simulink library "helperVarsizeLib"  (R2022b)
settings: Solver=VariableStepAuto  StartTime=0.0  StopTime=10.0  RelTol=1e-3
settings Model: Creator=The MathWorks, Inc.  LastModifiedBy=The MathWorks, Inc.
settings SolverCC: AlgebraicLoopSolver=TrustRegion
settings DebuggingCC: UnconnectedInputMsg=warning  UnconnectedOutputMsg=warning  UnconnectedLineMsg=warning  SFMachineParentedDataDiag=warning  ArithmeticOperatorsInVariantConditions=warning
settings ModelReferenceCC: EnableRefExpFcnMdlSchedulingChecks=on
settings SFSimCC: CustomCodeUndefinedFunction=UseInterfaceOnly
settings RTWCC: DLArmComputeVersion=19.05

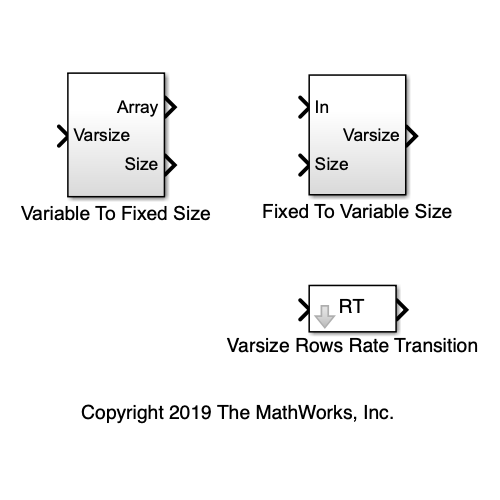
[thumbnail: Simulink's stored preview of the top-level diagram]
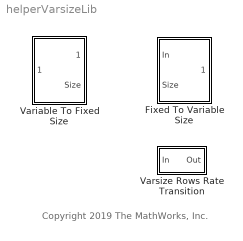
== system helperVarsizeLib ==
  note: Copyright 2019 The MathWorks, Inc.
  Fixed To Variable Size : Subsystem
  Variable To Fixed Size : Subsystem
  Varsize Rows Rate Transition : Subsystem  mask(Variable Size Rows Rate Transition){bufferInitialCondition=zeros(500,1)}
      mask prompts: bufferInitialCondition "Buffer initial condition"
      mask help: Helper block which enables rate transitions for arrays with variable sized rows. The maximium buffer size is the same as the buffer initial condition.
      mask Display: disp('RT')

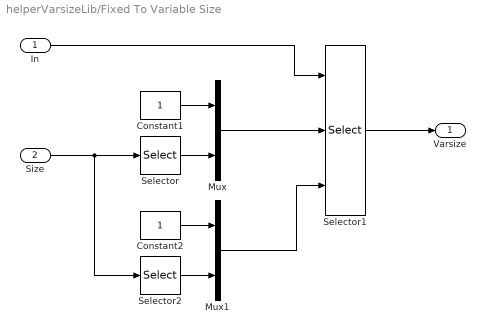
== system helperVarsizeLib/Fixed To Variable Size ==
  In : Inport
  Size : Inport  Port=2
  Constant1 : Constant  VectorParams1D=off
  Constant2 : Constant  VectorParams1D=off
  Mux : Mux  Inputs=2
  Mux1 : Mux  Inputs=2
  Selector : Selector  InputPortWidth=2  IndexOptions=Index vector (dialog)  Indices=1  OutputSizes=1
  Selector1 : Selector  NumberOfDimensions=2  InputPortWidth=3  IndexOptions=Starting and ending indices (port),Starting and ending indices (port)  Indices=[1 3],1  OutputSizes=1,1
  Selector2 : Selector  InputPortWidth=2  IndexOptions=Index vector (dialog)  Indices=2  OutputSizes=1
  Varsize : Outport  VectorParamsAs1DForOutWhenUnconnected=off
  wires:
  Constant2/1 -> Mux1/1
  Mux1/1 -> Selector1/3
  Selector2/1 -> Mux1/2
  Selector/1 -> Mux/2
  In/1 -> Selector1/1
  Selector1/1 -> Varsize/1
  Mux/1 -> Selector1/2
  Constant1/1 -> Mux/1
  Size/1 -> Selector/1, Selector2/1

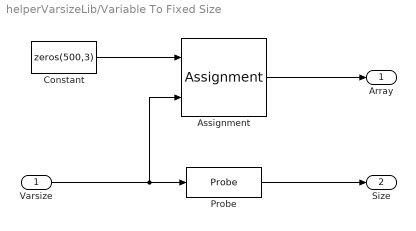
== system helperVarsizeLib/Variable To Fixed Size ==
  Varsize : Inport
  Assignment : Assignment  NumberOfDimensions=2  IndexMode=Zero-based  DiagnosticForDimensions=Warning  IndexOptions=Starting index (dialog),Starting index (dialog)  Indices=0,0  OutputSizes=1,1
  Constant : Constant  Value=zeros(500,3)  VectorParams1D=off
  Probe : Probe  ProbeWidth=off  ProbeSampleTime=off  ProbeComplexSignal=off  ProbeSignalDimensions=on
  Array : Outport  VectorParamsAs1DForOutWhenUnconnected=off
  Size : Outport  Port=2  VectorParamsAs1DForOutWhenUnconnected=off
  wires:
  Constant/1 -> Assignment/1
  Varsize/1 -> Probe/1, Assignment/2
  Assignment/1 -> Array/1
  Probe/1 -> Size/1

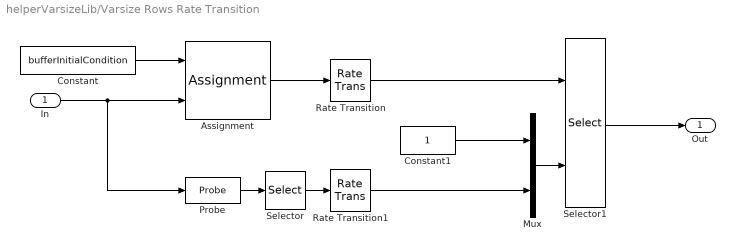
== system helperVarsizeLib/Varsize Rows Rate Transition ==
  In : Inport
  Assignment : Assignment  NumberOfDimensions=2  IndexMode=Zero-based  DiagnosticForDimensions=Warning  IndexOptions=Starting index (dialog),Starting index (dialog)  Indices=0,0  OutputSizes=1,1
  Constant : Constant  Value=bufferInitialCondition  VectorParams1D=off
  Constant1 : Constant  VectorParams1D=off
  Mux : Mux  Inputs=2
  Probe : Probe  ProbeWidth=off  ProbeSampleTime=off  ProbeComplexSignal=off  ProbeSignalDimensions=on
  Rate Transition : RateTransition  InitialCondition=bufferInitialCondition
  Rate Transition1 : RateTransition  InitialCondition=1
  Selector : Selector  InputPortWidth=2  IndexOptions=Index vector (dialog)  Indices=1  OutputSizes=1
  Selector1 : Selector  NumberOfDimensions=2  InputPortWidth=3  IndexOptions=Starting and ending indices (port),Select all  Indices=[1 3],1  OutputSizes=1,1
  Out : Outport  VectorParamsAs1DForOutWhenUnconnected=off
  wires:
  Selector/1 -> Rate Transition1/1
  In/1 -> Probe/1, Assignment/2
  Mux/1 -> Selector1/2
  Selector1/1 -> Out/1
  Assignment/1 -> Rate Transition/1
  Rate Transition/1 -> Selector1/1
  Constant1/1 -> Mux/1
  Constant/1 -> Assignment/1
  Probe/1 -> Selector/1
  Rate Transition1/1 -> Mux/2
